simulink model "simulate_quad_drone"  (R2019b)
settings: Solver=VariableStepAuto  StartTime=0.0  StopTime=120.0  RelTol=1e-3
PreLoadFcn:
  | set_param_quad;
undefined symbols (not defined in the file or in its folder): ParamQuad
settings Model: Creator=Bruno  LastModifiedBy=Nunes

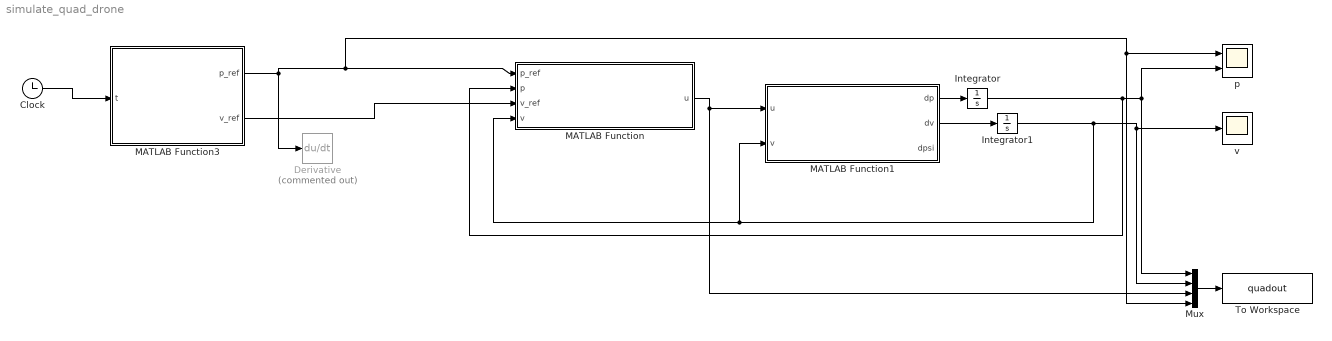
== system simulate_quad_drone ==
  Clock : Clock
  Derivative : Derivative  Commented=on
  Integrator : Integrator  InitialCondition=ParamQuad.p0
  Integrator1 : Integrator  InitialCondition=ParamQuad.v0
  MATLAB Function : MATLAB Function  TreatAsAtomicUnit=on
  MATLAB Function1 : MATLAB Function  TreatAsAtomicUnit=on
  MATLAB Function3 : MATLAB Function  TreatAsAtomicUnit=on
  Mux : Mux
  To Workspace : ToWorkspace  VariableName=quadout  SaveFormat=Timeseries  SampleTime=-1
  p : Scope  NumInputPorts=2
  "v " : Scope
  wires:
  MATLAB Function/1(u) -> MATLAB Function1/1(u), Mux/3
  MATLAB Function1/1(dp) -> Integrator/1
  MATLAB Function1/2(dv) -> Integrator1/1
  Integrator/1 -> p/2, Mux/1, MATLAB Function/2(p)
  Integrator1/1 -> Mux/2, "v "/1, MATLAB Function/4(v), MATLAB Function1/2(v)
  Mux/1 -> To Workspace/1
  Clock/1 -> MATLAB Function3/1(t)
  MATLAB Function3/1(p_ref) -> MATLAB Function/1(p_ref), Mux/4, p/1, Derivative/1
  MATLAB Function3/2(v_ref) -> MATLAB Function/3(v_ref)

== matlab function simulate_quad_drone/MATLAB Function1 ==
  data: u input; v input; dp output; dv output; ParamQuad parameter; dpsi output
function [dp,dv,dpsi] = drone_model(u,v,ParamQuad)
%DRONE_MODEL Summary of this function goes here
%   Detailed explanation goes here

 
    
    dp = v;
    dv = -[0;0;9.8] + 1/ParamQuad.m*u;
    dpsi = 0;
    
end

== matlab function simulate_quad_drone/MATLAB Function ==
  data: p_ref input; p input; v_ref input; u output; v input; ParamQuad parameter
function u = drone_controller(p_ref,p,v_ref,v,ParamQuad)
%DRONE_CONTROLLER Summary of this function goes here
%   Detailed explanation goes here

  
    
    u = -diag([ParamQuad.kp/2,ParamQuad.kp/2,ParamQuad.kp])*(p-p_ref) + ...
        -diag([ParamQuad.kv/2,ParamQuad.kv/2,ParamQuad.kv])*(v-v_ref) + [0;0;ParamQuad.m*9.8];
    
end

== matlab function simulate_quad_drone/MATLAB Function3 ==
  data: t input; p_ref output; v_ref output

function [p_ref , v_ref] = position_velocity_ref(t)


% if t < 30
%    p_ref = [sin(t);cos(t);3];
% else 
%     p_ref = [sin(t);cos(t);1];
% end



      
% if t < 20
%    p_ref = [1 + t/2; 1 ; 2];
%    
% elseif t > 20 & t < 40 
%    p_ref = [11+ cos(t) ; 2 + sin(t)  ;2 ];
%    %p_ref = [11 + cos(t); 2 +sin(t) ;2 ];
%    
% elseif t > 40 & t < 60 
%    p_ref = [ - t/2; 3 ;2 ];
%     
% else
%      p_ref = [0;0;0];     
%      
% end


%position
      
if t < 20
   p_ref = [ t/2; 0 ; 0.5];
   
elseif t > 20 & t < 80 

   p_ref = [ 10; 2 ; 0.5];
   
    
elseif t > 80 & t < 100 

   p_ref = [ 50 - t/2; 2 ;0.5 ];
else
     p_ref = [0;0;0.5];     
     
end


%velocity

if t < 20
   v_ref = [ 1/2; 0 ; 0];
   
elseif t > 20 & t < 80 

   v_ref = [ 0; 0 ;0 ];
 
elseif t > 80 & t < 100 

   v_ref = [  - 1/2; 0 ;0 ];
else
     v_ref = [0;0;0];     
     
end






end


%plot da trajectoria -  plot3(out.simout.Data(:,1), out.simout.Data(:,2), out.simout.Data(:,3));
